simulink model "E010A5_T2_trunc_one_inhibit_40A_1A_20260630"  (R2024b)
settings: Solver=VariableStepAuto  StartTime=0.0  StopTime=0.54e-3  MaxStep=5e-9  RelTol=1e-3
undefined symbols (not defined in the file): A_init, A_lower, A_upper, Cout, DCR_L1, DCR_L2, DCR_L3, DCR_L4, E010_AreaBleed_Enable, E010_AreaHold_Enable, E010_AreaHold_Time, E010_PulseInhibit_Count, E010_PulseInhibit_Enable, E010_PulseInhibit_Time, E010_Reentry_Band_Down, E010_ReentryGuard_Enable, E010_TonTrunc_Enable, E010_Vref, E010A5_DeltaI_Drop_Threshold_High, E010A5_IL_Sense_Gain1, E010A5_IL_Sense_Gain2, E010A5_IL_Sense_Gain3, E010A5_IL_Sense_Gain4, ESR_C, IdealIQCOT_Enable, IL_adc_counts_per_A, IL_pk_limit_adc_neg, IL_pk_limit_adc_pos, Iload_final, Iload_initial, Iph, Iqcot_enable, kappa_cmd, Kiqcot, Kvc_iqcot, L, Lambda0_iqcot, Lambda_m2, rho_cmd, Ri_iqcot, t_load_step, Tblank, Tdead, Tiqcot_leak, Toff_min, Ton_cmd, Ton_iq_max, Ton_iq_min, Ts_ctrl, Tslot, Tss, Tton_trunc_min, Tton_trunc_window, Vc_bias_iqcot, Vcot_ramp_amp, Vcot_ramp_enable, Vhys, Vin, Vo_ref
libraries: simulink x29, spsCurrentMeasurementLib x8, spsMosfetLib x8, spsSeriesRLCBranchLib x5, spsVoltageMeasurementLib x5, spsDCVoltageSourceLib x4, spsControlledCurrentSourceLib x1, spsGroundLib x1, spspowerguiLib x1
(part 2 of 2)

== system E010A5_T2_trunc_one_inhibit_40A_1A_20260630/GateDriver_1Phase1/OnDelay1 ==
  u : Inport
  Compare To Constant : simulink/Logic and Bit Operations/Compare To Constant  relop=>=  const=Tdead  OutDataTypeStr=boolean
  Data Type Conversion : DataTypeConversion  OutDataTypeStr=double  SaturateOnIntegerOverflow=off  RndMeth=Floor
  Integrator : Integrator  ExternalReset=level
  Logical Operator : Logic  Operator=NOT  AllPortsSameDT=off  OutDataTypeStr=boolean
  y : Outport
  wires:
  u/1 -> Data Type Conversion/1, Logical Operator/1
  Logical Operator/1 -> Integrator/2
  Data Type Conversion/1 -> Integrator/1
  Integrator/1 -> Compare To Constant/1
  Compare To Constant/1 -> y/1

== system E010A5_T2_trunc_one_inhibit_40A_1A_20260630/GateDriver_1Phase2/OnDelay ==
  u : Inport
  Compare To Constant : simulink/Logic and Bit Operations/Compare To Constant  relop=>=  const=Tdead  OutDataTypeStr=boolean
  Data Type Conversion : DataTypeConversion  OutDataTypeStr=double  SaturateOnIntegerOverflow=off  RndMeth=Floor
  Integrator : Integrator  ExternalReset=level
  Logical Operator : Logic  Operator=NOT  AllPortsSameDT=off  OutDataTypeStr=boolean
  y : Outport
  wires:
  u/1 -> Data Type Conversion/1, Logical Operator/1
  Logical Operator/1 -> Integrator/2
  Data Type Conversion/1 -> Integrator/1
  Integrator/1 -> Compare To Constant/1
  Compare To Constant/1 -> y/1

== system E010A5_T2_trunc_one_inhibit_40A_1A_20260630/GateDriver_1Phase2/OnDelay1 ==
  u : Inport
  Compare To Constant : simulink/Logic and Bit Operations/Compare To Constant  relop=>=  const=Tdead  OutDataTypeStr=boolean
  Data Type Conversion : DataTypeConversion  OutDataTypeStr=double  SaturateOnIntegerOverflow=off  RndMeth=Floor
  Integrator : Integrator  ExternalReset=level
  Logical Operator : Logic  Operator=NOT  AllPortsSameDT=off  OutDataTypeStr=boolean
  y : Outport
  wires:
  u/1 -> Data Type Conversion/1, Logical Operator/1
  Logical Operator/1 -> Integrator/2
  Data Type Conversion/1 -> Integrator/1
  Integrator/1 -> Compare To Constant/1
  Compare To Constant/1 -> y/1

== system E010A5_T2_trunc_one_inhibit_40A_1A_20260630/GateDriver_1Phase3/OnDelay ==
  u : Inport
  Compare To Constant : simulink/Logic and Bit Operations/Compare To Constant  relop=>=  const=Tdead  OutDataTypeStr=boolean
  Data Type Conversion : DataTypeConversion  OutDataTypeStr=double  SaturateOnIntegerOverflow=off  RndMeth=Floor
  Integrator : Integrator  ExternalReset=level
  Logical Operator : Logic  Operator=NOT  AllPortsSameDT=off  OutDataTypeStr=boolean
  y : Outport
  wires:
  u/1 -> Data Type Conversion/1, Logical Operator/1
  Logical Operator/1 -> Integrator/2
  Data Type Conversion/1 -> Integrator/1
  Integrator/1 -> Compare To Constant/1
  Compare To Constant/1 -> y/1

== system E010A5_T2_trunc_one_inhibit_40A_1A_20260630/GateDriver_1Phase3/OnDelay1 ==
  u : Inport
  Compare To Constant : simulink/Logic and Bit Operations/Compare To Constant  relop=>=  const=Tdead  OutDataTypeStr=boolean
  Data Type Conversion : DataTypeConversion  OutDataTypeStr=double  SaturateOnIntegerOverflow=off  RndMeth=Floor
  Integrator : Integrator  ExternalReset=level
  Logical Operator : Logic  Operator=NOT  AllPortsSameDT=off  OutDataTypeStr=boolean
  y : Outport
  wires:
  u/1 -> Data Type Conversion/1, Logical Operator/1
  Logical Operator/1 -> Integrator/2
  Data Type Conversion/1 -> Integrator/1
  Integrator/1 -> Compare To Constant/1
  Compare To Constant/1 -> y/1

== system E010A5_T2_trunc_one_inhibit_40A_1A_20260630/GateDriver_1Phase4/OnDelay ==
  u : Inport
  Compare To Constant : simulink/Logic and Bit Operations/Compare To Constant  relop=>=  const=Tdead  OutDataTypeStr=boolean
  Data Type Conversion : DataTypeConversion  OutDataTypeStr=double  SaturateOnIntegerOverflow=off  RndMeth=Floor
  Integrator : Integrator  ExternalReset=level
  Logical Operator : Logic  Operator=NOT  AllPortsSameDT=off  OutDataTypeStr=boolean
  y : Outport
  wires:
  u/1 -> Data Type Conversion/1, Logical Operator/1
  Logical Operator/1 -> Integrator/2
  Data Type Conversion/1 -> Integrator/1
  Integrator/1 -> Compare To Constant/1
  Compare To Constant/1 -> y/1

== system E010A5_T2_trunc_one_inhibit_40A_1A_20260630/GateDriver_1Phase4/OnDelay1 ==
  u : Inport
  Compare To Constant : simulink/Logic and Bit Operations/Compare To Constant  relop=>=  const=Tdead  OutDataTypeStr=boolean
  Data Type Conversion : DataTypeConversion  OutDataTypeStr=double  SaturateOnIntegerOverflow=off  RndMeth=Floor
  Integrator : Integrator  ExternalReset=level
  Logical Operator : Logic  Operator=NOT  AllPortsSameDT=off  OutDataTypeStr=boolean
  y : Outport
  wires:
  u/1 -> Data Type Conversion/1, Logical Operator/1
  Logical Operator/1 -> Integrator/2
  Data Type Conversion/1 -> Integrator/1
  Integrator/1 -> Compare To Constant/1
  Compare To Constant/1 -> y/1

== matlab function E010A5_T2_trunc_one_inhibit_40A_1A_20260630/E010A5_TonTrunc3 ==
  data: ton_in input double size=1; ton_out output double size=1; t input double size=1; t_step input double size=1; t_window input double size=1; t_min input double size=1; enable input double size=1; trunc_active output double size=1; ton_saved output double size=1
function [ton_out,trunc_active,ton_saved] = ton_trunc(ton_in,t,t_step,t_window,t_min,enable)
%#codegen
active = (enable > 0.5) && (t >= t_step) && (t <= (t_step + t_window));
if active
    ton_out = min(ton_in, t_min);
else
    ton_out = ton_in;
end
trunc_active = double(active);
ton_saved = max(ton_in - ton_out, 0.0);

== matlab function E010A5_T2_trunc_one_inhibit_40A_1A_20260630/E010A5_TonTrunc4 ==
  data: ton_in input double size=1; ton_out output double size=1; t input double size=1; t_step input double size=1; t_window input double size=1; t_min input double size=1; enable input double size=1; trunc_active output double size=1; ton_saved output double size=1
function [ton_out,trunc_active,ton_saved] = ton_trunc(ton_in,t,t_step,t_window,t_min,enable)
%#codegen
active = (enable > 0.5) && (t >= t_step) && (t <= (t_step + t_window));
if active
    ton_out = min(ton_in, t_min);
else
    ton_out = ton_in;
end
trunc_active = double(active);
ton_saved = max(ton_in - ton_out, 0.0);

== matlab function E010A5_T2_trunc_one_inhibit_40A_1A_20260630/E010A5_PulseInhibitState ==
  data: u1 input boolean size=1; y output double size=1; u2 input boolean size=1; u3 input boolean size=1; u4 input boolean size=1
function y = any_four(u1,u2,u3,u4)
%#codegen
y = double((u1 > 0.5) || (u2 > 0.5) || (u3 > 0.5) || (u4 > 0.5));

== matlab function E010A5_T2_trunc_one_inhibit_40A_1A_20260630/E010A5_PulseInhibit1 ==
  data: tr_in input boolean size=1; tr_out output boolean size=1; t input double size=1; t_step input double size=1; t_window input double size=1; count_max input double size=1; enable input double size=1; vout input double size=1; vref input double size=1; reentry_band input double size=1; guard_enable input double size=1; inhibit_active output boolean size=1; inhibit_count output double size=1
function [tr_out,inhibit_active,inhibit_count] = pulse_inhibit(tr_in,t,t_step,t_window,count_max,enable,vout,vref,reentry_band,guard_enable)
%#codegen
is_high = logical(tr_in);
in_window = (enable > 0.5) && (t >= t_step) && (t <= (t_step + t_window));
guard_ok = (guard_enable <= 0.5) || (vout >= (vref + reentry_band));
inhibit_active = is_high && in_window && (count_max > 0.0) && guard_ok;
if inhibit_active
    tr_out = false;
else
    tr_out = tr_in;
end
inhibit_count = double(inhibit_active);

== matlab function E010A5_T2_trunc_one_inhibit_40A_1A_20260630/E010A5_PulseInhibit2 ==
  data: tr_in input boolean size=1; tr_out output boolean size=1; t input double size=1; t_step input double size=1; t_window input double size=1; count_max input double size=1; enable input double size=1; vout input double size=1; vref input double size=1; reentry_band input double size=1; guard_enable input double size=1; inhibit_active output boolean size=1; inhibit_count output double size=1
function [tr_out,inhibit_active,inhibit_count] = pulse_inhibit(tr_in,t,t_step,t_window,count_max,enable,vout,vref,reentry_band,guard_enable)
%#codegen
is_high = logical(tr_in);
in_window = (enable > 0.5) && (t >= t_step) && (t <= (t_step + t_window));
guard_ok = (guard_enable <= 0.5) || (vout >= (vref + reentry_band));
inhibit_active = is_high && in_window && (count_max > 0.0) && guard_ok;
if inhibit_active
    tr_out = false;
else
    tr_out = tr_in;
end
inhibit_count = double(inhibit_active);

== matlab function E010A5_T2_trunc_one_inhibit_40A_1A_20260630/E010A5_PulseInhibit3 ==
  data: tr_in input boolean size=1; tr_out output boolean size=1; t input double size=1; t_step input double size=1; t_window input double size=1; count_max input double size=1; enable input double size=1; vout input double size=1; vref input double size=1; reentry_band input double size=1; guard_enable input double size=1; inhibit_active output boolean size=1; inhibit_count output double size=1
function [tr_out,inhibit_active,inhibit_count] = pulse_inhibit(tr_in,t,t_step,t_window,count_max,enable,vout,vref,reentry_band,guard_enable)
%#codegen
is_high = logical(tr_in);
in_window = (enable > 0.5) && (t >= t_step) && (t <= (t_step + t_window));
guard_ok = (guard_enable <= 0.5) || (vout >= (vref + reentry_band));
inhibit_active = is_high && in_window && (count_max > 0.0) && guard_ok;
if inhibit_active
    tr_out = false;
else
    tr_out = tr_in;
end
inhibit_count = double(inhibit_active);

== matlab function E010A5_T2_trunc_one_inhibit_40A_1A_20260630/E010A5_PulseInhibit4 ==
  data: tr_in input boolean size=1; tr_out output boolean size=1; t input double size=1; t_step input double size=1; t_window input double size=1; count_max input double size=1; enable input double size=1; vout input double size=1; vref input double size=1; reentry_band input double size=1; guard_enable input double size=1; inhibit_active output boolean size=1; inhibit_count output double size=1
function [tr_out,inhibit_active,inhibit_count] = pulse_inhibit(tr_in,t,t_step,t_window,count_max,enable,vout,vref,reentry_band,guard_enable)
%#codegen
is_high = logical(tr_in);
in_window = (enable > 0.5) && (t >= t_step) && (t <= (t_step + t_window));
guard_ok = (guard_enable <= 0.5) || (vout >= (vref + reentry_band));
inhibit_active = is_high && in_window && (count_max > 0.0) && guard_ok;
if inhibit_active
    tr_out = false;
else
    tr_out = tr_in;
end
inhibit_count = double(inhibit_active);

== matlab function E010A5_T2_trunc_one_inhibit_40A_1A_20260630/E010A5_AreaHold_EnableProjection ==
  data: enable_in input double size=1; enable_out output double size=1; t input double size=1; t_step input double size=1; t_hold input double size=1; hold_enable input double size=1; vout input double size=1; vref input double size=1; reentry_band input double size=1; bleed_enable input double size=1; hold_state output double size=1; hold_count output double size=1; reset_count output double size=1; bleed_count output double size=1; reentry_state output double size=1
function [enable_out,hold_state,hold_count,reset_count,bleed_count,reentry_state] = area_hold_enable(enable_in,t,t_step,t_hold,hold_enable,vout,vref,reentry_band,bleed_enable)
%#codegen
persistent was_hold reset_seen
if isempty(was_hold)
    was_hold = false;
end
if isempty(reset_seen)
    reset_seen = 0.0;
end
if t < t_step
    was_hold = false;
    reset_seen = 0.0;
end
in_window = (hold_enable > 0.5) && (t >= t_step) && (t <= (t_step + t_hold));
release_not_safe = vout >= (vref + reentry_band);
hold = in_window && release_not_safe;
enable_out = double(enable_in > 0.5);
if hold
    enable_out = 0.0;
end
hold_state = double(hold);
hold_count = double(hold);
bleed_count = double(hold && (bleed_enable > 0.5));
release_edge = (~hold) && was_hold;
if release_edge
    reset_seen = reset_seen + 1.0;
end
reset_count = reset_seen;
reentry_state = double((hold_enable > 0.5) && (t > t_step) && ~hold);
was_hold = hold;

== matlab function E010A5_T2_trunc_one_inhibit_40A_1A_20260630/E010A5_REQRejectReason ==
  data: r1 input boolean size=1; reason output double size=1; r2 input boolean size=1; r3 input boolean size=1; r4 input boolean size=1; a1 input boolean size=1; a2 input boolean size=1; a3 input boolean size=1; a4 input boolean size=1
function reason = req_reject_reason(r1,r2,r3,r4,a1,a2,a3,a4)
%#codegen
raw = (r1 > 0.5) || (r2 > 0.5) || (r3 > 0.5) || (r4 > 0.5);
acc = (a1 > 0.5) || (a2 > 0.5) || (a3 > 0.5) || (a4 > 0.5);
if raw && ~acc
    reason = 1.0;
else
    reason = 0.0;
end

== matlab function E010A5_T2_trunc_one_inhibit_40A_1A_20260630/E010A5_PhaseOrderError ==
  data: a1 input boolean size=1; err output double size=1; a2 input boolean size=1; a3 input boolean size=1; a4 input boolean size=1; t input double size=1; t_step input double size=1
function err = phase_order_error(a1,a2,a3,a4,t,t_step)
%#codegen
persistent prev expected
if isempty(prev)
    prev = [false,false,false,false];
end
if isempty(expected)
    expected = 0.0;
end
acc = [a1,a2,a3,a4] > 0.5;
rise = acc & ~prev;
err = 0.0;
if t < t_step
    expected = 0.0;
else
    for idx = 1:4
        if rise(idx)
            if expected > 0.5 && double(idx) ~= expected
                err = 1.0;
            end
            expected = double(idx + 1);
            if expected > 4.0
                expected = 1.0;
            end
        end
    end
end
prev = acc;

== matlab function E010A5_T2_trunc_one_inhibit_40A_1A_20260630/E010A5_SevereDropDetector ==
  data: iload input double size=1; detected output double size=1; t input double size=1; threshold input double size=1
function detected = severe_drop_detector(iload,t,threshold)
%#codegen
persistent initial_load latched
if isempty(initial_load)
    initial_load = iload;
end
if isempty(latched)
    latched = false;
end
if t < 1.0e-9
    initial_load = iload;
    latched = false;
end
if (initial_load - iload) >= threshold
    latched = true;
end
detected = double(latched);

== matlab function E010A5_T2_trunc_one_inhibit_40A_1A_20260630/E010A5_TonActual1 ==
  data: qh input boolean size=1; Ton_actual output double size=1; t input double size=1
function Ton_actual = ton_actual_estimator(qh, t)
%#codegen
persistent q_prev t_rise last_width
if isempty(q_prev)
    q_prev = 0.0;
end
if isempty(t_rise)
    t_rise = 0.0;
end
if isempty(last_width)
    last_width = 0.0;
end
is_high = double(qh > 0.5);
if is_high > 0.5 && q_prev <= 0.5
    t_rise = t;
elseif is_high <= 0.5 && q_prev > 0.5
    last_width = max(0.0, t - t_rise);
end
Ton_actual = last_width;
q_prev = is_high;

== matlab function E010A5_T2_trunc_one_inhibit_40A_1A_20260630/E010A5_TonActual2 ==
  data: qh input boolean size=1; Ton_actual output double size=1; t input double size=1
function Ton_actual = ton_actual_estimator(qh, t)
%#codegen
persistent q_prev t_rise last_width
if isempty(q_prev)
    q_prev = 0.0;
end
if isempty(t_rise)
    t_rise = 0.0;
end
if isempty(last_width)
    last_width = 0.0;
end
is_high = double(qh > 0.5);
if is_high > 0.5 && q_prev <= 0.5
    t_rise = t;
elseif is_high <= 0.5 && q_prev > 0.5
    last_width = max(0.0, t - t_rise);
end
Ton_actual = last_width;
q_prev = is_high;

== matlab function E010A5_T2_trunc_one_inhibit_40A_1A_20260630/E010A5_TonActual3 ==
  data: qh input boolean size=1; Ton_actual output double size=1; t input double size=1
function Ton_actual = ton_actual_estimator(qh, t)
%#codegen
persistent q_prev t_rise last_width
if isempty(q_prev)
    q_prev = 0.0;
end
if isempty(t_rise)
    t_rise = 0.0;
end
if isempty(last_width)
    last_width = 0.0;
end
is_high = double(qh > 0.5);
if is_high > 0.5 && q_prev <= 0.5
    t_rise = t;
elseif is_high <= 0.5 && q_prev > 0.5
    last_width = max(0.0, t - t_rise);
end
Ton_actual = last_width;
q_prev = is_high;

== matlab function E010A5_T2_trunc_one_inhibit_40A_1A_20260630/E010A5_TonActual4 ==
  data: qh input boolean size=1; Ton_actual output double size=1; t input double size=1
function Ton_actual = ton_actual_estimator(qh, t)
%#codegen
persistent q_prev t_rise last_width
if isempty(q_prev)
    q_prev = 0.0;
end
if isempty(t_rise)
    t_rise = 0.0;
end
if isempty(last_width)
    last_width = 0.0;
end
is_high = double(qh > 0.5);
if is_high > 0.5 && q_prev <= 0.5
    t_rise = t;
elseif is_high <= 0.5 && q_prev > 0.5
    last_width = max(0.0, t - t_rise);
end
Ton_actual = last_width;
q_prev = is_high;

== matlab function E010A5_T2_trunc_one_inhibit_40A_1A_20260630/E010A5_ActiveHSPhase ==
  data: qh1 input boolean size=1; active_phase output double size=1; qh2 input boolean size=1; qh3 input boolean size=1; qh4 input boolean size=1
function active_phase = active_hs_phase(qh1,qh2,qh3,qh4)
%#codegen
qh = [qh1, qh2, qh3, qh4] > 0.5;
active_phase = 0.0;
for idx = 1:4
    if qh(idx)
        active_phase = double(idx);
        return;
    end
end

== matlab function E010A5_T2_trunc_one_inhibit_40A_1A_20260630/Ideal_Digital_IQCOT_Request/IQCOT_Event_Core ==
  data: e_v input double size=1; REQ_iqcot output double size=1; IL1 input double size=1; IL2 input double size=1; IL3 input double size=1; IL4 input double size=1; phase_idx input double size=1; tr_reset input double size=1; enable input double size=1; Ts_ctrl_in input double size=1; Lambda0_in input double size=1; Lambda_m2_in input double size=1; rho_cmd_in input double size=1; Ri_in input double size=1; Kvc_in input double size=1; Vc_bias_in input double size=1; kappa_cmd_in input double size=1; A_init_in input double size=1; A_lower_in input double size=1; A_upper_in input double size=1; A_iqcot output double size=1; Lambda_i output double size=1; h_iqcot output double size=1; IL_sel output double size=1; vc_ctrl output double size=1
function [REQ_iqcot,A_iqcot,Lambda_i,h_iqcot,IL_sel,vc_ctrl] = IQCOT_Event_Core(e_v,IL1,IL2,IL3,IL4,phase_idx,tr_reset,enable,Ts_ctrl_in,Lambda0_in,Lambda_m2_in,rho_cmd_in,Ri_in,Kvc_in,Vc_bias_in,kappa_cmd_in,A_init_in,A_lower_in,A_upper_in)
%#codegen
REQ_iqcot = 0.0;
A_iqcot = 0.0;
Lambda_i = 0.0;
h_iqcot = 0.0;
IL_sel = 0.0;
vc_ctrl = 0.0;
persistent Astate reset_prev phase_prev
if isempty(Astate)
    Astate = double(A_init_in);
end
if isempty(reset_prev)
    reset_prev = 0.0;
end
if isempty(phase_prev)
    phase_prev = 0.0;
end
p = floor(double(phase_idx));
p = mod(p, 4);
if p == 0
    IL_sel = IL1;
elseif p == 1
    IL_sel = IL2;
elseif p == 2
    IL_sel = IL3;
else
    IL_sel = IL4;
end
Ri_eff = Ri_in * exp(kappa_cmd_in);
vc_ctrl = Vc_bias_in + Kvc_in * e_v;
h_iqcot = vc_ctrl - Ri_eff * IL_sel;
Lambda_i = Lambda0_in * (1 + rho_cmd_in) + Lambda_m2_in * cos(pi * p);
if Lambda_i < eps
    Lambda_i = eps;
end
A_update = Astate + Ts_ctrl_in * h_iqcot;
if A_update < A_lower_in
    A_update = A_lower_in;
end
if A_update > A_upper_in
    A_update = A_upper_in;
end
REQ_iqcot = double((enable > 0.5) && (A_update >= Lambda_i));
A_iqcot = A_update;
reset_rise = (tr_reset > 0.5) && (reset_prev <= 0.5);
phase_change = (p ~= phase_prev);
if enable <= 0.5
    Astate = A_init_in;
elseif reset_rise || phase_change
    Astate = A_init_in;
else
    Astate = A_update;
end
reset_prev = double(tr_reset);
phase_prev = p;

== matlab function E010A5_T2_trunc_one_inhibit_40A_1A_20260630/E010A5_CurrentLimitHit ==
  data: u1 input boolean size=1; y output double size=1; u2 input boolean size=1; u3 input boolean size=1; u4 input boolean size=1
function y = any_four(u1,u2,u3,u4)
%#codegen
y = double((u1 > 0.5) || (u2 > 0.5) || (u3 > 0.5) || (u4 > 0.5));

== matlab function E010A5_T2_trunc_one_inhibit_40A_1A_20260630/E010A5_TonTrunc1 ==
  data: ton_in input double size=1; ton_out output double size=1; t input double size=1; t_step input double size=1; t_window input double size=1; t_min input double size=1; enable input double size=1; trunc_active output double size=1; ton_saved output double size=1
function [ton_out,trunc_active,ton_saved] = ton_trunc(ton_in,t,t_step,t_window,t_min,enable)
%#codegen
active = (enable > 0.5) && (t >= t_step) && (t <= (t_step + t_window));
if active
    ton_out = min(ton_in, t_min);
else
    ton_out = ton_in;
end
trunc_active = double(active);
ton_saved = max(ton_in - ton_out, 0.0);

== matlab function E010A5_T2_trunc_one_inhibit_40A_1A_20260630/E010A5_TonTrunc2 ==
  data: ton_in input double size=1; ton_out output double size=1; t input double size=1; t_step input double size=1; t_window input double size=1; t_min input double size=1; enable input double size=1; trunc_active output double size=1; ton_saved output double size=1
function [ton_out,trunc_active,ton_saved] = ton_trunc(ton_in,t,t_step,t_window,t_min,enable)
%#codegen
active = (enable > 0.5) && (t >= t_step) && (t <= (t_step + t_window));
if active
    ton_out = min(ton_in, t_min);
else
    ton_out = ton_in;
end
trunc_active = double(active);
ton_saved = max(ton_in - ton_out, 0.0);
